simulink model "Fault_Test"  (R2022b)
settings: Solver=FixedStepDiscrete  StartTime=0.0  StopTime=10.0  FixedStep=0.5  RelTol=1e-3
undefined symbols (not defined in the file): sigbuilder_block
settings Model: Creator=ZYH  LastModifiedBy=ZYH

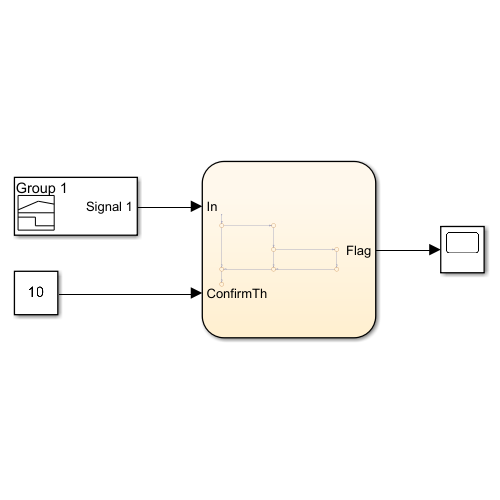
[thumbnail: Simulink's stored preview of the top-level diagram]
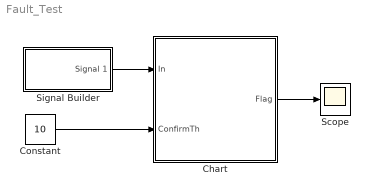
== system Fault_Test ==
  Chart : Stateflow chart  TreatAsAtomicUnit=on
  Constant : Constant  Value=10
  Scope : Scope
  Signal Builder : Subsystem  Tag=STV Subsys  LoadFcn=sigbuilder_block('load',[437.6 199.2 550.4 400 ]);  StartFcn=sigbuilder_block('start');  StopFcn=sigbuilder_block('stop');  ClipboardFcn=sigbuilder_block('clipboard');  mask(Sigbuilder block){tuvar=[0:10]}
      mask help: Simulink:masks:SigbuilderBlock_MD
      mask init:
      | if ~strcmp(get_param(bdroot(gcbh),'SimulationStatus'),'stopped') tuvar = sigbuilder_block('maskInit'); end
      settings: CopyFcn=sigbuilder_block('copy');  DeleteFcn=sigbuilder_block('delete');  ModelCloseFcn=sigbuilder_block('modelClose');  PreSaveFcn=sigbuilder_block('preSave');  PauseFcn=sigbuilder_block('pause');  ContinueFcn=sigbuilder_block('continue');  NameChangeFcn=sigbuilder_block('namechange');  OpenFcn=sigbuilder_block('open',[437.6 199.2 550.4 400 ]);  CloseFcn=sigbuilder_block('close');
      mask Display: plot(0, 0, 100, 100,[2, 2, 32, 32, 2], [68, 8, 8, 68, 68],[32, 2], [38, 38], [32, 19, 2],[53, 60, 44], [32, 17, 17, 2],[16, 16, 31, 31]);txt = getActiveGroup(gcbh);text(2, 100, txt,'verticalAlignment', 'top');
  wires:
  Signal Builder/1(Signal 1) -> Chart/1(In)
  Constant/1 -> Chart/2(ConfirmTh)
  Chart/1(Flag) -> Scope/1

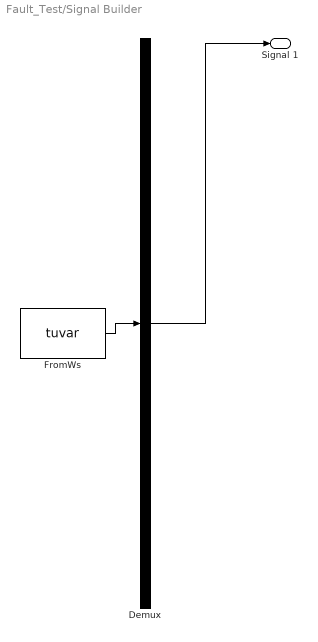
== system Fault_Test/Signal Builder ==
  Demux : Demux  Tag=STV Demux  Outputs=1
      settings: DisplayOption=none
  FromWs : FromWorkspace  Tag=STV FromWs  VariableName=tuvar
      SigBuilderData=|
      | common.afterFinalStr = 'Extrapolate'
      | common.sampleTime = 0
      | dataSet.timeRange = [0 10]
      | dataSet.name = 'Group 1'
      | sbobj.Groups.Name = 'Group 1'
      | sbobj.Groups.Signals.Name = 'Signal 1'
      | sbobj.Groups.Signals.XData = [0 6 6 10]
      | sbobj.Groups.Signals.YData = [1 1 0 0]
  Signal 1 : Outport  Tag=STV Outport
  wires:
  Demux/1 -> Signal 1/1
  FromWs/1 -> Demux/1

== stateflow chart Fault_Test/Chart ==
  (default) -> (junction 2)
  (junction 2) -> (junction 4) [order 1] : [In == true]
  (junction 2) -> (junction 18) [order 2]
  (junction 4) -> (junction 6) : {Cnt = Cnt+1}
  (junction 6) -> (junction 11) [order 1] : [Cnt > ConfirmTh]
  (junction 6) -> (junction 15) [order 2]
  (junction 11) -> (junction 13) : {Flag = true;
      | Cnt = 0;}
  (junction 15) -> (junction 18)
  (junction 13) -> (junction 15)
  (junction 18) -> (junction 21)
  data: In input; Cnt local =0; ConfirmTh input; Flag output
